simulink model "eric_idea_matlab_function_working"  (R2022b)
settings: Solver=VariableStepAuto  StartTime=0.0  StopTime=inf  RelTol=1e-3
libraries: slrealtimeiplib x2
settings Model: Creator=operator  LastModifiedBy=operator

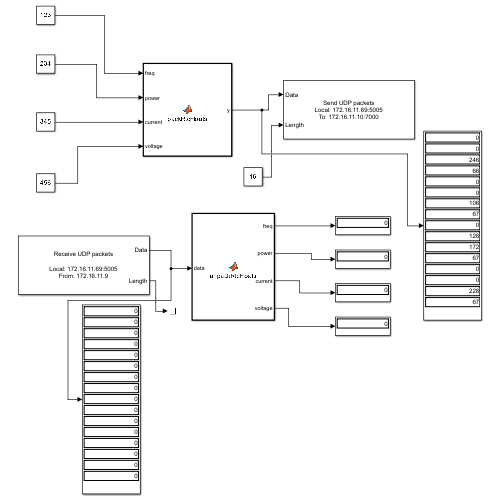
[thumbnail: Simulink's stored preview of the top-level diagram]
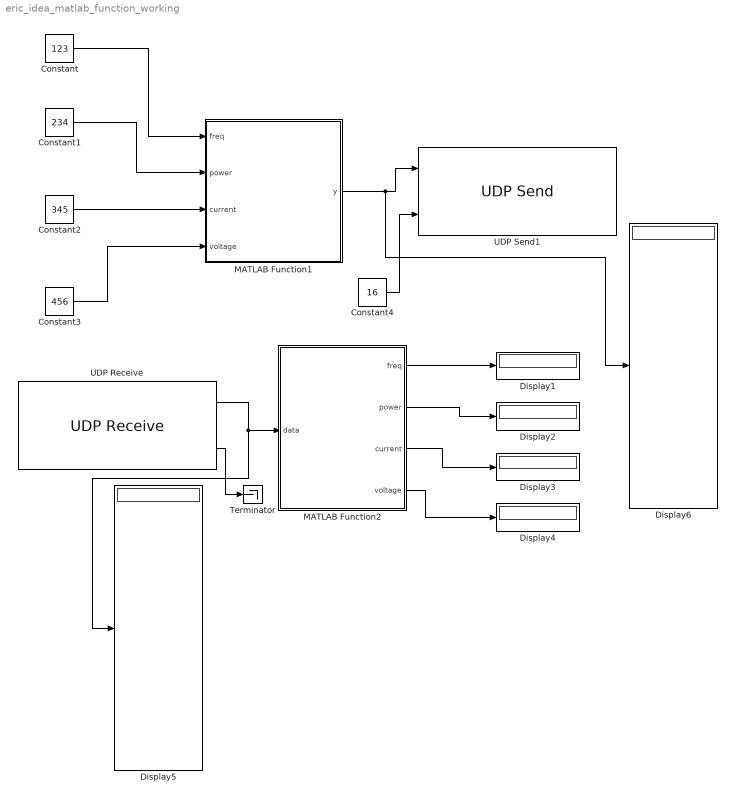
== system eric_idea_matlab_function_working ==
  Constant : Constant  Value=123  OutDataTypeStr=double
  Constant1 : Constant  Value=234  OutDataTypeStr=double
  Constant2 : Constant  Value=345  OutDataTypeStr=double
  Constant3 : Constant  Value=456  OutDataTypeStr=double
  Constant4 : Constant  Value=16
  Display{1..6} (6 alike) : Display
  MATLAB Function1 : MATLAB Function  TreatAsAtomicUnit=on
  MATLAB Function2 : MATLAB Function  TreatAsAtomicUnit=on
  Terminator : Terminator
  UDP Receive : slrealtimeiplib/UDP Receive  useHostTargetConn=off  ipAddress=172.16.11.69  localPort=5005  rcvWidth=16  rcvFmAny=off  fmAddress=172.16.11.9  sampleTime=0.01  enableMessage=off  maxPackets=1
  UDP Send1 : slrealtimeiplib/UDP Send  useHostTargetConn=off  toAddress=172.16.11.10  toPort=7000  sampleTime=0.1  enableMessage=off  ipAddress=172.16.11.69  localPort=5005
  wires:
  Constant/1 -> MATLAB Function1/1(freq)
  Constant1/1 -> MATLAB Function1/2(power)
  Constant2/1 -> MATLAB Function1/3(current)
  Constant3/1 -> MATLAB Function1/4(voltage)
  MATLAB Function1/1(y) -> Display6/1, UDP Send1/1
  Constant4/1 -> UDP Send1/2
  UDP Receive/2 -> Terminator/1
  MATLAB Function2/4(voltage) -> Display4/1
  MATLAB Function2/3(current) -> Display3/1
  MATLAB Function2/2(power) -> Display2/1
  MATLAB Function2/1(freq) -> Display1/1
  UDP Receive/1 -> Display5/1, MATLAB Function2/1(data)

== matlab function eric_idea_matlab_function_working/MATLAB Function1 ==
  data: freq input double size=1; y output uint8 size=[1 16]; power input double size=1; current input double size=1; voltage input double size=1
function y = packRtcFloats(freq, power, current, voltage)
    %#codegen
    % Inputs: freq, power, current, voltage (double)
    % Output: y (1x16 uint8)
    coder.varsize('y', [1 16], [0 0]);
    y = zeros(1, 16, 'uint8');
    
    % Debug: Log input values (codegen-compatible)
    coder.ceval('printf', 'Packing freq: %f, power: %f, current: %f, voltage: %f\n', freq, power, current, voltage);
    
    y = [typecast(single(freq), 'uint8'), ...
         typecast(single(power), 'uint8'), ...
         typecast(single(current), 'uint8'), ...
         typecast(single(voltage), 'uint8')];
end

== matlab function eric_idea_matlab_function_working/MATLAB Function2 ==
  data: data input uint8 size=[1 16]; freq output double size=1; power output double size=1; current output double size=1; voltage output double size=1
 % old function : sending to .10 and receiving from .10 after echo from
 % mqtt to udp
% function [freq, power, current, voltage] = unpackRtcFloats(data)
    %#codegen
    % Input: data (1x16 uint8)
    % Outputs: freq, power, current, voltage (double)
    %  coder.varsize('data', [1 16], [0 0]);
  %    if length(data) == 16
    %      floatData = typecast(uint8(data), 'single');
    %      freq = double(floatData(1));    % Convert to double for output
    %      power = double(floatData(2));   % Convert to double for output
    %      current = double(floatData(3)); % Convert to double for output
     %     voltage = double(floatData(4)); % Convert to double for output
  %    else
  %        freq = 0;
   %       power = 0;
    %      current = 0;
     %     voltage = 0;
    %      disp('Warning: Invalid data length, expected 16 bytes.');
  %    end
 % end
  

  % new function to excho in client to broker
  function [freq, power, current, voltage] = unpackRtcFloats(data)
    %#codegen
    coder.varsize('data', [1 16], [0 0]);
    
    if length(data) == 16
        coder.ceval('printf', 'Input data length: 16\n');
        for i = 1:16
            coder.ceval('printf', 'Byte %d: %d\n', i-1, data(i));
        end
        
        byteMatrix = reshape(data, [4, 4])';
        floatData = swapbytes(typecast(byteMatrix(:), 'single')); % Add swapbytes for big-endian
        freq = double(floatData(1));
        power = double(floatData(2));
        current = double(floatData(3));
        voltage = double(floatData(4));
    else
        coder.ceval('printf', 'Input data length: %d, expected 16\n', length(data));
        freq = 0.0;
        power = 0.0;
        current = 0.0;
        voltage = 0.0;
    end
end
